simulink model "host_leading"  (R2020b)
settings: Solver=VariableStepAuto  StartTime=0.0  StopTime=60.0  RelTol=1e-3
model workspace: external: MAT-File /Users/alessandro/Desktop/AdaptiveCC/alenicco.mat (data not in the file)
values from neighbouring files (symbols this model uses):
  d_0 = 8    [ACC.m]
  Kd_err = 0.2    [ACC.m]
  Kv = 0.5    [ACC.m]
  Kv_r = 0.4    [ACC.m]
  t_h_tar = 1    [ACC.m]
  v_h = 28    [ACC.m]
  v_l = 36    [ACC.m]
  v_tar = 36    [ACC.m]
  x_h = 0    [ACC.m]
  x_l = 50    [ACC.m]
libraries: simulink x4
settings Model: OrderedModelArguments=off  Creator=alessandro  LastModifiedBy=gabriele

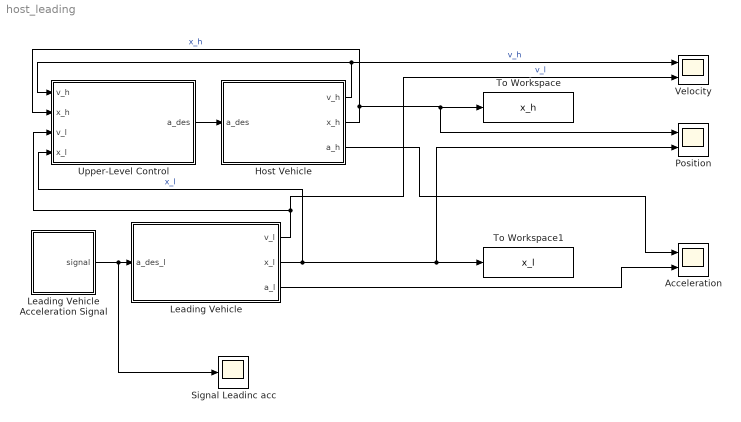
== system host_leading ==
  Acceleration : Scope  NumInputPorts=2
  "Host Vehicle " : Subsystem  Tag=host vehicle
  "Leading Vehicle " : Subsystem
  Leading Vehicle Acceleration Signal : Subsystem
  Position : Scope  NumInputPorts=2
  Signal Leadinc acc : Scope
  To Workspace : ToWorkspace  VariableName=x_h  SampleTime=-1
  To Workspace1 : ToWorkspace  VariableName=x_l  SampleTime=-1
  Upper-Level Control : Subsystem
  Velocity : Scope  NumInputPorts=2
  wires:
  "Leading Vehicle "/2(x_l) -> Position/2, To Workspace1/1, Upper-Level Control/4(x_l)  "x_l"
  "Host Vehicle "/1(v_h) -> Velocity/1, Upper-Level Control/1(v_h)  "v_h"
  "Host Vehicle "/2("x_h ") -> Upper-Level Control/2(x_h), Position/1, To Workspace/1  "x_h"
  Upper-Level Control/1(a_des) -> "Host Vehicle "/1(a_des)
  Leading Vehicle Acceleration Signal/1(signal) -> Signal Leadinc acc/1, "Leading Vehicle "/1(a_des_l)
  "Leading Vehicle "/1(v_l) -> Velocity/2, Upper-Level Control/3(v_l)  "v_l"
  "Host Vehicle "/3(a_h) -> Acceleration/1
  "Leading Vehicle "/3(a_l) -> Acceleration/2

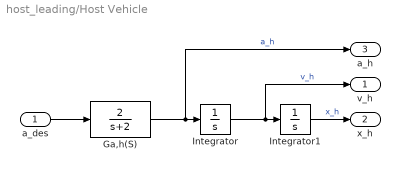
== system host_leading/Host Vehicle  ==
  a_des : Inport
  Ga,h(S) : TransferFcn  Numerator=[2]  Denominator=[1 2]
  Integrator : Integrator  InitialCondition=v_h
  Integrator1 : Integrator  InitialCondition=x_h
  v_h : Outport
  "x_h " : Outport  Port=2
  a_h : Outport  Port=3
  wires:
  Integrator/1 -> Integrator1/1, v_h/1  "v_h"
  Ga,h(S)/1 -> a_h/1, Integrator/1  "a_h"
  a_des/1 -> Ga,h(S)/1
  Integrator1/1 -> "x_h "/1  "x_h"

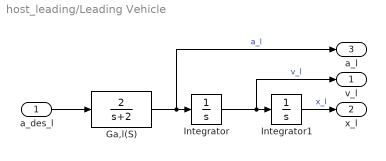
== system host_leading/Leading Vehicle  ==
  a_des_l : Inport
  Ga,l(S) : TransferFcn  Numerator=[2]  Denominator=[1 2]
  Integrator : Integrator  InitialCondition=v_l
  Integrator1 : Integrator  InitialCondition=x_l
  v_l : Outport
  x_l : Outport  Port=2
  a_l : Outport  Port=3
  wires:
  Integrator/1 -> v_l/1, Integrator1/1  "v_l"
  Integrator1/1 -> x_l/1  "x_l"
  Ga,l(S)/1 -> a_l/1, Integrator/1  "a_l"
  a_des_l/1 -> Ga,l(S)/1

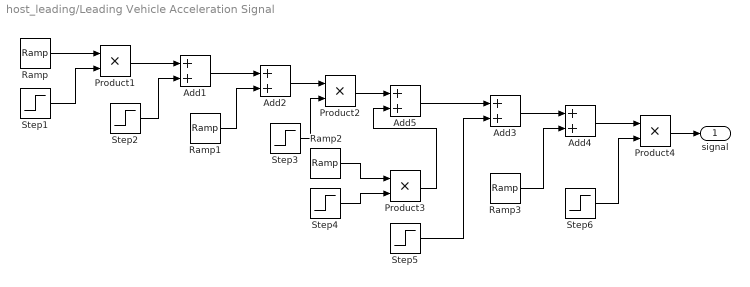
== system host_leading/Leading Vehicle Acceleration Signal ==
  Add{1..5} (5 alike) : Sum
  Product{1..4} (4 alike) : Product
  Ramp : simulink/Sources/Ramp  slope=-4  start=10  InitialOutput=0
  Ramp1 : simulink/Sources/Ramp  slope=4  start=13.5  InitialOutput=0
  Ramp2 : simulink/Sources/Ramp  slope=4  start=40  InitialOutput=0
  Ramp3 : simulink/Sources/Ramp  slope=-4  start=43.5  InitialOutput=0
  Step1 : Step  Time=10.5  Before=1  After=0  SampleTime=0.1
  Step2 : Step  Time=10.5  After=-2  SampleTime=0
  Step3 : Step  Time=14  Before=1  After=0  SampleTime=0
  Step4 : Step  Time=40.5  Before=1  After=0  SampleTime=0
  Step5 : Step  Time=40.5  After=2  SampleTime=0
  Step6 : Step  Time=44  Before=1  After=0  SampleTime=0
  signal : Outport
  wires:
  Product4/1 -> signal/1
  Add1/1 -> Add2/1
  Step3/1 -> Product2/2
  Product3/1 -> Add5/2
  Step5/1 -> Add3/2
  Add2/1 -> Product2/1
  Step1/1 -> Product1/2
  Product2/1 -> Add5/1
  Step2/1 -> Add1/2
  Ramp2/1 -> Product3/1
  Product1/1 -> Add1/1
  Add4/1 -> Product4/1
  Ramp/1 -> Product1/1
  Add3/1 -> Add4/1
  Step6/1 -> Product4/2
  Ramp1/1 -> Add2/2
  Step4/1 -> Product3/2
  Add5/1 -> Add3/1
  Ramp3/1 -> Add4/2

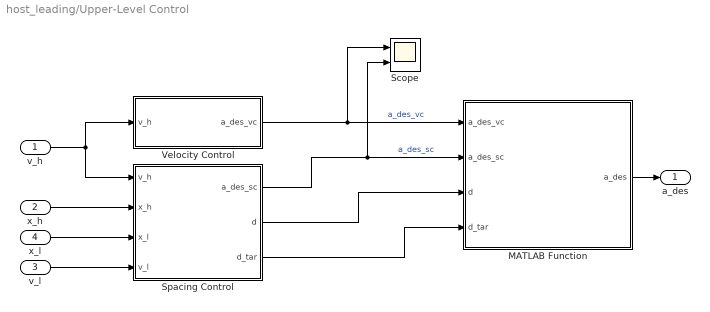
== system host_leading/Upper-Level Control ==
  v_h : Inport
  x_h : Inport  Port=2
  v_l : Inport  Port=3
  x_l : Inport  Port=4
  MATLAB Function : MATLAB Function  TreatAsAtomicUnit=on
  Scope : Scope  NumInputPorts=2
  Spacing Control : Subsystem
  Velocity Control : Subsystem
  a_des : Outport
  wires:
  Spacing Control/1(a_des_sc) -> Scope/2, MATLAB Function/2(a_des_sc)  "a_des_sc"
  Velocity Control/1(a_des_vc) -> Scope/1, MATLAB Function/1(a_des_vc)  "a_des_vc"
  v_l/1 -> Spacing Control/4(v_l)
  x_l/1 -> Spacing Control/3(x_l)
  Spacing Control/2(d) -> MATLAB Function/3(d)
  Spacing Control/3(d_tar) -> MATLAB Function/4(d_tar)
  MATLAB Function/1(a_des) -> a_des/1
  x_h/1 -> Spacing Control/2(x_h)
  v_h/1 -> Velocity Control/1(v_h), Spacing Control/1(v_h)

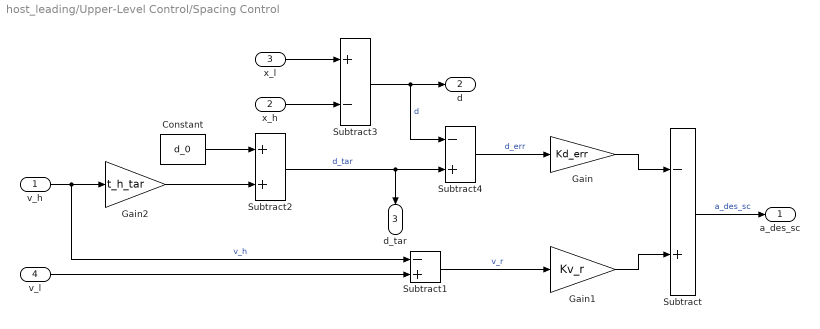
== system host_leading/Upper-Level Control/Spacing Control ==
  v_h : Inport
  x_h : Inport  Port=2
  x_l : Inport  Port=3
  v_l : Inport  Port=4
  Constant : Constant  Value=d_0
  Gain : Gain  Gain=Kd_err
  Gain1 : Gain  Gain=Kv_r
  Gain2 : Gain  Gain=t_h_tar
  Subtract : Sum  Inputs=-+
  Subtract1 : Sum  Inputs=-+
  Subtract2 : Sum
  Subtract3 : Sum  Inputs=+-
  Subtract4 : Sum  Inputs=-+
  a_des_sc : Outport
  d : Outport  Port=2
  d_tar : Outport  Port=3
  wires:
  Gain/1 -> Subtract/1
  Gain1/1 -> Subtract/2
  Subtract/1 -> a_des_sc/1  "a_des_sc"
  v_h/1 -> Subtract1/1, Gain2/1  "v_h"
  Subtract1/1 -> Gain1/1  "v_r"
  Gain2/1 -> Subtract2/2
  v_l/1 -> Subtract1/2
  x_l/1 -> Subtract3/1
  x_h/1 -> Subtract3/2
  Subtract2/1 -> Subtract4/2, d_tar/1  "d_tar"
  Subtract3/1 -> Subtract4/1, d/1  "d"
  Subtract4/1 -> Gain/1  "d_err"
  Constant/1 -> Subtract2/1

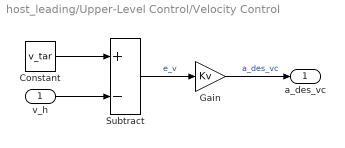
== system host_leading/Upper-Level Control/Velocity Control ==
  v_h : Inport
  Constant : Constant  Value=v_tar
  Gain : Gain  Gain=Kv
  Subtract : Sum  Inputs=+-
  a_des_vc : Outport
  wires:
  v_h/1 -> Subtract/2
  Constant/1 -> Subtract/1
  Subtract/1 -> Gain/1  "e_v"
  Gain/1 -> a_des_vc/1  "a_des_vc"

== matlab function host_leading/Upper-Level Control/MATLAB Function ==
  data: a_des_vc input; a_des output; a_des_sc input; d input; d_tar input
function a_des = switching_logic(a_des_vc, a_des_sc, d, d_tar)

if d > d_tar
    a_des = min([a_des_vc a_des_sc]);
else
    a_des = a_des_sc;
end

if a_des > 5 
    a_des = 5;
end

if a_des < -3
    a_des = -3;
end


end
